simulink model "main"  (R2025b)
settings: Solver=VariableStepAuto  StartTime=0.0  StopTime=10.0  RelTol=1e-3
model workspace (MAT data in the model file):
  CMD = 3
settings Model: Creator=00091  LastModifiedBy=00091

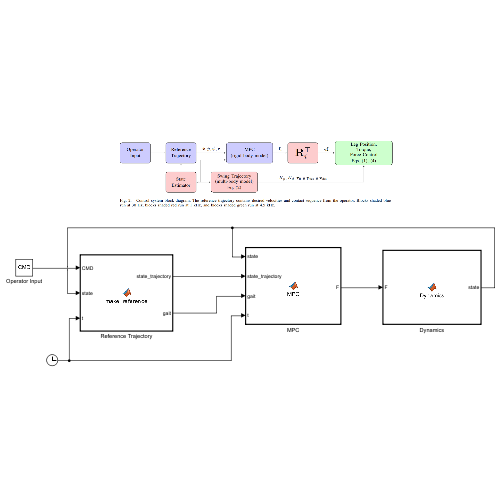
[thumbnail: Simulink's stored preview of the top-level diagram]
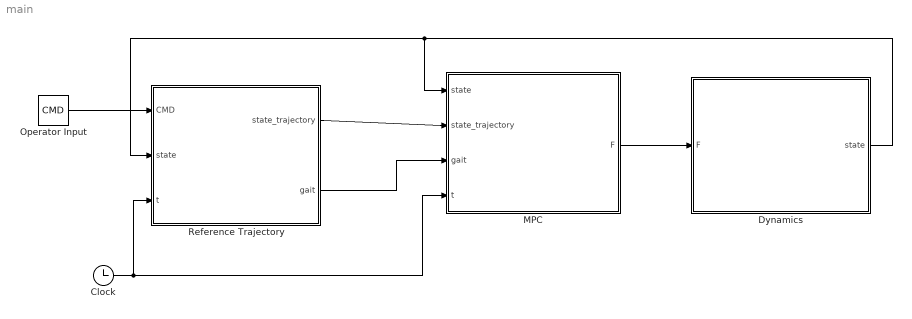
== system main ==
  Clock : Clock
  Dynamics : MATLAB Function  TreatAsAtomicUnit=on
  MPC : MATLAB Function  TreatAsAtomicUnit=on
  Operator Input : Constant  Value=CMD
  Reference Trajectory : MATLAB Function  TreatAsAtomicUnit=on
  wires:
  Operator Input/1 -> Reference Trajectory/1(CMD)
  Dynamics/1(state) -> MPC/1(state), Reference Trajectory/2(state)
  Reference Trajectory/1(state_trajectory) -> MPC/2(state_trajectory)
  MPC/1(F) -> Dynamics/1(F)
  Reference Trajectory/2(gait) -> MPC/3(gait)
  Clock/1 -> MPC/4(t), Reference Trajectory/3(t)

== matlab function main/MPC ==
  data: state input; state_trajectory input; gait input; F output; t input
function F = MPC(state, state_trajectory, gait, t)

F = u;

== matlab function main/Reference Trajectory ==
  data: CMD input; state_trajectory output; state input; gait output; t input
function [state_trajectory, gait]= make_reference(CMD, state, t)

state_trajectory, gait = u;

== matlab function main/Dynamics ==
  data: F input; state output
function state= Dynamics(F)

state = u;
